simulink model "Q2P4"  (Simulink 6.3)
settings: Solver=ode45  StartTime=0.0  StopTime=10  RelTol=1e-3
libraries: simulink x2
settings Model: LastModifiedBy=Frank Gloria  StrictBusMsg=None
settings OptimizationCC: InlineInvariantSignals=on

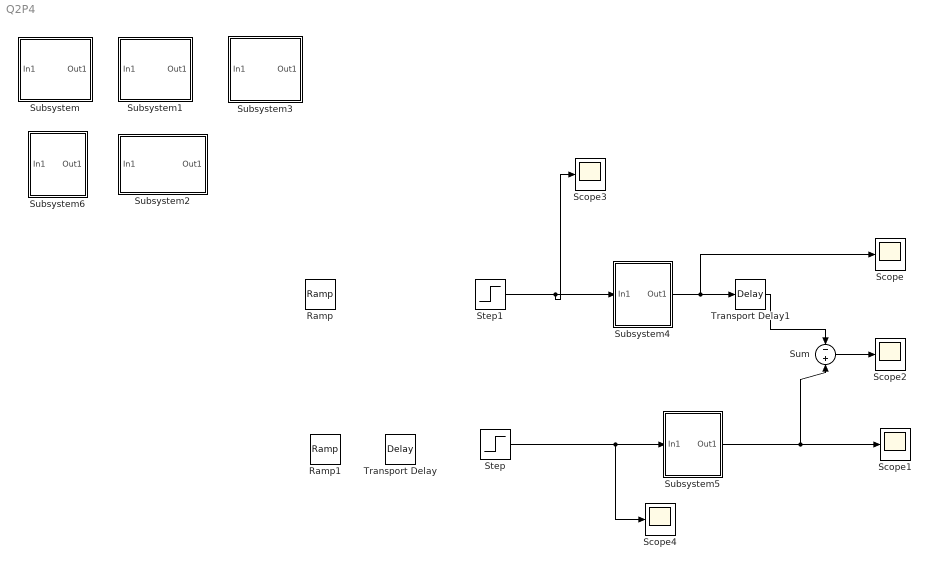
== system Q2P4 ==
  Ramp : simulink/Sources/Ramp  slope=1  start=0  X0=0
  Ramp1 : simulink/Sources/Ramp  slope=1  start=0  X0=0
  Scope{,1..4} (5 alike) : Scope
      Scope2 settings: SaveName=ScopeData2
      Scope3 settings: SaveName=ScopeData3
      Scope4 settings: SaveName=ScopeData4
  Step : Step  Time=3  SampleTime=0
  Step1 : Step  Time=0  Before=1  SampleTime=0
  Subsystem : Subsystem
      mask Display: disp('Planta P1')
  Subsystem1 : Subsystem
      mask Display: disp('Planta P2')
  Subsystem2 : Subsystem
      mask Display: disp('Planta P5')
  Subsystem3 : Subsystem
      mask Display: disp('Planta P3')
  Subsystem4 : Subsystem
      mask Display: disp('Planta P4')
  Subsystem5 : Subsystem
      mask Display: disp('Planta P4')
  Subsystem6 : Subsystem
      mask Display: disp('Planta P4')
  Sum : Sum  Inputs=-+
  Transport Delay : TransportDelay  DelayTime=3
  Transport Delay1 : TransportDelay  DelayTime=3
  wires:
  Subsystem5/1(Out1) -> Scope1/1, Sum/2
  Sum/1 -> Scope2/1
  Transport Delay1/1 -> Sum/1
  Step1/1 -> Scope3/1, Subsystem4/1(In1)
  Step/1 -> Scope4/1, Subsystem5/1(In1)
  Subsystem4/1(Out1) -> Transport Delay1/1, Scope/1

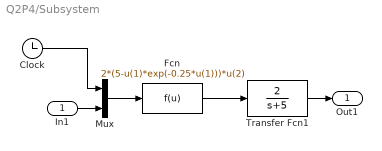
== system Q2P4/Subsystem ==
  In1 : Inport
  Clock : Clock
      settings: Decimation=10
  Fcn : Fcn  Expr=2*(5-u(1)*exp(-0.25*u(1)))*u(2)
  Mux : Mux  Inputs=2
  Transfer Fcn1 : TransferFcn  Numerator=[2]  Denominator=[1 5]
  Out1 : Outport
  wires:
  Clock/1 -> Mux/1
  Mux/1 -> Fcn/1
  Fcn/1 -> Transfer Fcn1/1
  Transfer Fcn1/1 -> Out1/1
  In1/1 -> Mux/2

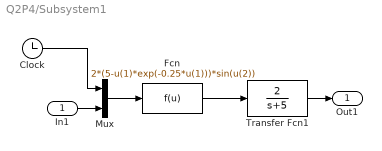
== system Q2P4/Subsystem1 ==
  In1 : Inport
  Clock : Clock
      settings: Decimation=10
  Fcn : Fcn  Expr=2*(5-u(1)*exp(-0.25*u(1)))*sin(u(2))
  Mux : Mux  Inputs=2
  Transfer Fcn1 : TransferFcn  Numerator=[2]  Denominator=[1 5]
  Out1 : Outport
  wires:
  Clock/1 -> Mux/1
  Mux/1 -> Fcn/1
  Fcn/1 -> Transfer Fcn1/1
  Transfer Fcn1/1 -> Out1/1
  In1/1 -> Mux/2

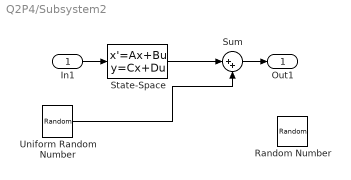
== system Q2P4/Subsystem2 ==
  In1 : Inport
  Random Number : RandomNumber  Variance=0.25  SampleTime=0
  State-Space : StateSpace  A=[-1 -2;1 0]  B=[1; 0]  C="[0  2]"  D=0
  Sum : Sum  Inputs=|++
  Uniform Random Number : UniformRandomNumber  Minimum=-0.25  Maximum=0.25  SampleTime=0
  Out1 : Outport
  wires:
  State-Space/1 -> Sum/1
  In1/1 -> State-Space/1
  Sum/1 -> Out1/1
  Uniform Random Number/1 -> Sum/2

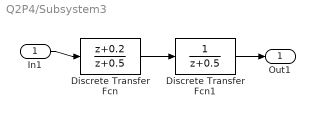
== system Q2P4/Subsystem3 ==
  In1 : Inport
  Discrete Transfer Fcn : DiscreteTransferFcn  Numerator=[1 0.2]
  Discrete Transfer Fcn1 : DiscreteTransferFcn
  Out1 : Outport
  wires:
  Discrete Transfer Fcn/1 -> Discrete Transfer Fcn1/1
  Discrete Transfer Fcn1/1 -> Out1/1
  In1/1 -> Discrete Transfer Fcn/1

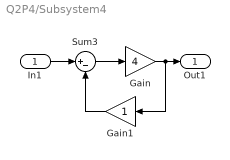
== system Q2P4/Subsystem4 ==
  In1 : Inport
  Gain : Gain  Gain=4
  Gain1 : Gain  Orientation=left
  Sum3 : Sum  Inputs=|+-
  Out1 : Outport
  wires:
  Sum3/1 -> Gain/1
  Gain1/1 -> Sum3/2
  Gain/1 -> Out1/1, Gain1/1
  In1/1 -> Sum3/1

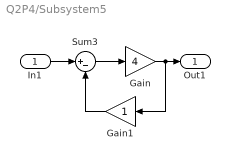
== system Q2P4/Subsystem5 ==
  In1 : Inport
  Gain : Gain  Gain=4
  Gain1 : Gain  Orientation=left
  Sum3 : Sum  Inputs=|+-
  Out1 : Outport
  wires:
  Sum3/1 -> Gain/1
  Gain1/1 -> Sum3/2
  Gain/1 -> Out1/1, Gain1/1
  In1/1 -> Sum3/1

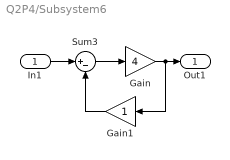
== system Q2P4/Subsystem6 ==
  In1 : Inport
  Gain : Gain  Gain=4
  Gain1 : Gain  Orientation=left
  Sum3 : Sum  Inputs=|+-
  Out1 : Outport
  wires:
  Sum3/1 -> Gain/1
  Gain1/1 -> Sum3/2
  Gain/1 -> Out1/1, Gain1/1
  In1/1 -> Sum3/1
